simulink model "Grid_modelling_Thermal_V7_ALfix_sheddable_ramped"  (R2025b)
settings: Solver=ode45  StopTime=5000  MaxStep=0.01
libraries: simulink x20, slpidlib x10
(part 1 of 3)
settings Model: Creator=ASUS  LastModifiedBy=naren

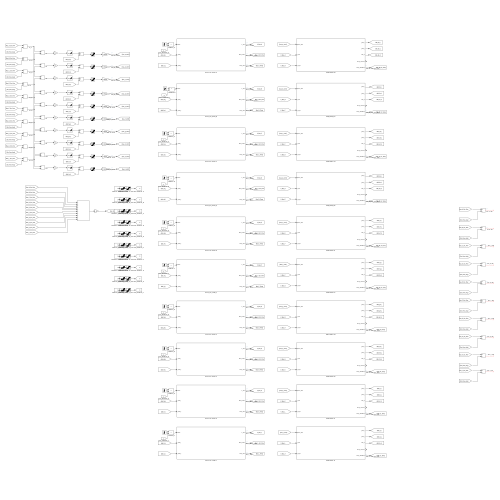
[thumbnail: Simulink's stored preview of the top-level diagram]
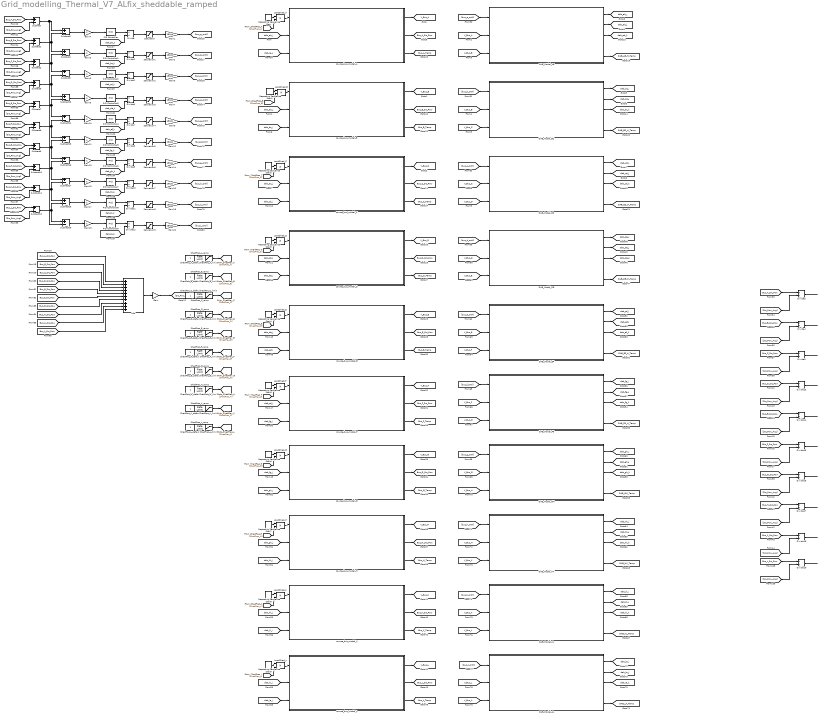
== system Grid_modelling_Thermal_V7_ALfix_sheddable_ramped ==
  Add : Sum  Inputs=++++++++++
  DAB_Model_AB : Subsystem
  DAB_Model_AL : Subsystem
  DAB_Model_BC : Subsystem
  DAB_Model_CD : Subsystem
  DAB_Model_DE : Subsystem
  DAB_Model_EF : Subsystem
  DAB_Model_FG : Subsystem
  DAB_Model_GH : Subsystem
  DAB_Model_HK : Subsystem
  DAB_Model_KL : Subsystem
  Divide{,1..19} (20 alike) : Product  Inputs=*/
  Gain : Gain  Gain=1/10
  Gain{1..3,7,9,12,14,16,18,20} (10 alike) : Gain  Gain=180/pi
  Gain{4..6,8,10..11,13,15,17,19} (10 alike) : Gain  Gain=-1
  LoadShed_A : Product
  LoadShed_B : Product
  LoadShed_C : Product
  LoadShed_D : Product
  LoadShed_E : Product
  LoadShed_F : Product
  LoadShed_G : Product
  LoadShed_H : Product
  LoadShed_K : Product
  LoadShed_L : Product
  PID Controller{,1..9} (10 alike) : slpidlib/PID Controller  Controller=PI  Form=Parallel  TimeDomain=Discrete-time  UseExternalTs=off  SampleTime=0.01  IntegratorMethod=Forward Euler  FilterMethod=Forward Euler  ControllerParametersSource=internal  P=0.2  I=0.1  UseKiTs=off  D=0  UseExternalDerivativeSource=off  N=100  UseFilter=on  TunerSelectOption=Transfer Function Based (PID Tuner App)  InitialConditionSource=internal  InitialConditionForIntegrator=0  InitialConditionForFilter=0  DifferentiatorICPrevScaledInput=0  ExternalReset=none  TrackingMode=off  Kt=1  LimitOutput=on  SatLimitsSource=internal  UpperSaturationLimit=100e3  LowerSaturationLimit=-100e3  LinearizeAsGain=on  AntiWindupMode=none  Kb=1  LimitIntegrator=off  UpperIntegratorSaturationLimit=inf  LowerIntegratorSaturationLimit=-inf  POutMin=[]  POutMax=[]  IOutMin=[]  IOutMax=[]  DOutMin=[]  DOutMax=[]  NOutMin=[]  NOutMax=[]  SumOutMin=[]  SumOutMax=[]  SaturationOutMin=[]  SaturationOutMax=[]  PParamMin=[]  PParamMax=[]  IParamMin=[]  IParamMax=[]  DParamMin=[]  DParamMax=[]  NParamMin=[]  NParamMax=[]  KbParamMin=[]  KbParamMax=[]  KtParamMin=[]  KtParamMax=[]  KbOutMin=[]  KbOutMax=[]  KtOutMin=[]  KtOutMax=[]  IntegratorOutMin=[]  IntegratorOutMax=[]  FilterOutMin=[]  FilterOutMax=[]  SumI1OutMin=[]  SumI1OutMax=[]  SumI2OutMin=[]  SumI2OutMax=[]  SumI3OutMin=[]  SumI3OutMax=[]  SumI4OutMin=[]  SumI4OutMax=[]  SumDOutMin=[]  SumDOutMax=[]  DifferentiatorOutMin=[]  DifferentiatorOutMax=[]  FilterDiffOutCoefMin=[]  FilterDiffOutCoefMax=[]  ReciprocalOutMin=[]  ReciprocalOutMax=[]  SumDenOutMin=[]  SumDenOutMax=[]  SumNumOutMin=[]  SumNumOutMax=[]  DivideOutMin=[]  DivideOutMax=[]  UdiffTsProdOutMin=[]  UdiffTsProdOutMax=[]  NTsProdOutMin=[]  NTsProdOutMax=[]  UintegralTsProdOutMin=[]  UintegralTsProdOutMax=[]  UngainTsProdOutMin=[]  UngainTsProdOutMax=[]  ClampingZeroOutDataTypeStr=Inherit: Inherit via back propagation  ClampingZeroOutMin=[]  ClampingZeroOutMax=[]  FilterDenConstantOutDataTypeStr=Inherit: Inherit via back propagation  FilterDenConstantOutMin=[]  FilterDenConstantOutMax=[]  PCopyOutDataTypeStr=Inherit: Inherit via back propagation  PCopyOutMin=[]  PCopyOutMax=[]  NCopyOutDataTypeStr=Inherit: Inherit via back propagation  NCopyOutMin=[]  NCopyOutMax=[]  IntegratorContinuousStateAttributes=''  IntegratorStateMustResolveToSignalObject=off  IntegratorRTWStateStorageClass=Auto  FilterContinuousStateAttributes=''  FilterStateMustResolveToSignalObject=off  FilterRTWStateStorageClass=Auto  ParallelPVariant=InternalParameters  IdealPVariant=Disabled  IVariant=InternalParameters  DVariant=Disabled  IntegratorVariant=Discrete  SatVariant=Enabled  AWVariant=Passthrough  PCopyVariant=Disabled  TRVariant=Disabled  FdbkBlocksVariant=Forward  IdealPFdbkVariant=Disabled  SatFdbkVariant=Disabled  DerivativeFilterVariant=Disabled  NVariant=Disabled  NCopyVariant=Disabled_SignalSpec  FilterICVariant=Disabled  IntegratorICVariant=InternalICs  ExternalResetVariant=Disabled  TRSumVariant=Passthrough  SumFdbkVariant=Disabled  SumVariant=Sum_PI  TsampFilterVariant=InternalTs  TsampNgainVariant=Passthrough  TsampIntegralVariant=Disabled_SignalSpec  ExternalSaturationOutDataTypeStr=Inherit: Same as second input  DerivativeSourceVariant=Disabled  PreIntVariant=InternalPreInt
  Repeating Sequence Stair : simulink/Sources/Repeating Sequence Stair  OutValues=Pload_A.'  tsamp=0.01  OutMin=[]  OutMax=[]  OutDataTypeStr=double  OutputDataTypeScalingMode=double  OutDataType=fixdt(0,8)  ConRadixGroup=Best Precision: Vector-wise  OutScaling=2^-12
  Repeating Sequence Stair1 : simulink/Sources/Repeating Sequence Stair  OutValues=Pload_B.'  tsamp=0.01  OutMin=[]  OutMax=[]  OutDataTypeStr=double  OutputDataTypeScalingMode=double  OutDataType=fixdt(0,8)  ConRadixGroup=Best Precision: Vector-wise  OutScaling=2^-12
  Repeating Sequence Stair2 : simulink/Sources/Repeating Sequence Stair  OutValues=Pload_C.'  tsamp=0.01  OutMin=[]  OutMax=[]  OutDataTypeStr=double  OutputDataTypeScalingMode=double  OutDataType=fixdt(0,8)  ConRadixGroup=Best Precision: Vector-wise  OutScaling=2^-12
  Repeating Sequence Stair3 : simulink/Sources/Repeating Sequence Stair  OutValues=Pload_D.'  tsamp=0.01  OutMin=[]  OutMax=[]  OutDataTypeStr=double  OutputDataTypeScalingMode=double  OutDataType=fixdt(0,8)  ConRadixGroup=Best Precision: Vector-wise  OutScaling=2^-12
  Repeating Sequence Stair4 : simulink/Sources/Repeating Sequence Stair  OutValues=Pload_E.'  tsamp=0.01  OutMin=[]  OutMax=[]  OutDataTypeStr=double  OutputDataTypeScalingMode=double  OutDataType=fixdt(0,8)  ConRadixGroup=Best Precision: Vector-wise  OutScaling=2^-12
  Repeating Sequence Stair5 : simulink/Sources/Repeating Sequence Stair  OutValues=Pload_F.'  tsamp=0.01  OutMin=[]  OutMax=[]  OutDataTypeStr=double  OutputDataTypeScalingMode=double  OutDataType=fixdt(0,8)  ConRadixGroup=Best Precision: Vector-wise  OutScaling=2^-12
  Repeating Sequence Stair6 : simulink/Sources/Repeating Sequence Stair  OutValues=Pload_G.'  tsamp=0.01  OutMin=[]  OutMax=[]  OutDataTypeStr=double  OutputDataTypeScalingMode=double  OutDataType=fixdt(0,8)  ConRadixGroup=Best Precision: Vector-wise  OutScaling=2^-12
  Repeating Sequence Stair7 : simulink/Sources/Repeating Sequence Stair  OutValues=Pload_H.'  tsamp=0.01  OutMin=[]  OutMax=[]  OutDataTypeStr=double  OutputDataTypeScalingMode=double  OutDataType=fixdt(0,8)  ConRadixGroup=Best Precision: Vector-wise  OutScaling=2^-12
  Repeating Sequence Stair8 : simulink/Sources/Repeating Sequence Stair  OutValues=Pload_K.'  tsamp=0.01  OutMin=[]  OutMax=[]  OutDataTypeStr=double  OutputDataTypeScalingMode=double  OutDataType=fixdt(0,8)  ConRadixGroup=Best Precision: Vector-wise  OutScaling=2^-12
  Repeating Sequence Stair9 : simulink/Sources/Repeating Sequence Stair  OutValues=Pload_L.'  tsamp=0.01  OutMin=[]  OutMax=[]  OutDataTypeStr=double  OutputDataTypeScalingMode=double  OutDataType=fixdt(0,8)  ConRadixGroup=Best Precision: Vector-wise  OutScaling=2^-12
  Saturation{,1..9} (10 alike) : Saturate  UpperLimit=pi/2  LowerLimit=-pi/2
  ShedFrac_A_default : Constant
  ShedFrac_A_limit : Saturate  UpperLimit=1  LowerLimit=0
  ShedFrac_A_ramp : RateLimiter  RisingSlewLimit=inf  FallingSlewLimit=-inf  SampleTimeMode=inherited
  ShedFrac_B_default : Constant
  ShedFrac_B_limit : Saturate  UpperLimit=1  LowerLimit=0
  ShedFrac_B_ramp : RateLimiter  RisingSlewLimit=inf  FallingSlewLimit=-inf  SampleTimeMode=inherited
  ShedFrac_C_default : Constant
  ShedFrac_C_limit : Saturate  UpperLimit=1  LowerLimit=0
  ShedFrac_C_ramp : RateLimiter  RisingSlewLimit=inf  FallingSlewLimit=-inf  SampleTimeMode=inherited
  ShedFrac_D_default : Constant
  ShedFrac_D_limit : Saturate  UpperLimit=1  LowerLimit=0
  ShedFrac_D_ramp : RateLimiter  RisingSlewLimit=inf  FallingSlewLimit=-inf  SampleTimeMode=inherited
  ShedFrac_E_default : Constant
  ShedFrac_E_limit : Saturate  UpperLimit=1  LowerLimit=0
  ShedFrac_E_ramp : RateLimiter  RisingSlewLimit=inf  FallingSlewLimit=-inf  SampleTimeMode=inherited
  ShedFrac_F_default : Constant
  ShedFrac_F_limit : Saturate  UpperLimit=1  LowerLimit=0
  ShedFrac_F_ramp : RateLimiter  RisingSlewLimit=inf  FallingSlewLimit=-inf  SampleTimeMode=inherited
  ShedFrac_G_default : Constant
  ShedFrac_G_limit : Saturate  UpperLimit=1  LowerLimit=0
  ShedFrac_G_ramp : RateLimiter  RisingSlewLimit=inf  FallingSlewLimit=-inf  SampleTimeMode=inherited
  ShedFrac_H_default : Constant
  ShedFrac_H_limit : Saturate  UpperLimit=1  LowerLimit=0
  ShedFrac_H_ramp : RateLimiter  RisingSlewLimit=inf  FallingSlewLimit=-inf  SampleTimeMode=inherited
  ShedFrac_K_default : Constant
  ShedFrac_K_limit : Saturate  UpperLimit=1  LowerLimit=0
  ShedFrac_K_ramp : RateLimiter  RisingSlewLimit=inf  FallingSlewLimit=-inf  SampleTimeMode=inherited
  ShedFrac_L_default : Constant
  ShedFrac_L_limit : Saturate  UpperLimit=1  LowerLimit=0
  ShedFrac_L_ramp : RateLimiter  RisingSlewLimit=inf  FallingSlewLimit=-inf  SampleTimeMode=inherited
  Subtract{,1..19} (20 alike) : Sum  Inputs=+-
  source_bus_model_A : Subsystem
  source_bus_model_B : Subsystem
  source_bus_model_C : Subsystem
  source_bus_model_D : Subsystem
  source_bus_model_E : Subsystem
  source_bus_model_F : Subsystem
  source_bus_model_G : Subsystem
  source_bus_model_H : Subsystem
  source_bus_model_K : Subsystem
  source_bus_model_L : Subsystem
  tag scope: Bus_A_Src_Pow=global, Bus_A_Temp=global, Bus_B_Src_Pow=global, Bus_B_Temp=global, Bus_C_Src_Pow=global, Bus_C_Temp=global, Bus_D_Src_Pow=global, Bus_D_Temp=global, Bus_E_Src_Pow=global, Bus_E_Temp=global, Bus_F_Src_Pow=global, Bus_F_Temp=global, Bus_G_Src_Pow=global, Bus_G_Temp=global, Bus_H_Src_Pow=global, Bus_H_Temp=global, Bus_K_Src_Pow=global, Bus_K_Temp=global, Bus_L_Src_Pow=global, Bus_L_Temp=global, DAB_AB_H_Temp=global, DAB_BC_H_Temp=global, DAB_CD_H_Temp=global, DAB_DE_H_Temp=global, DAB_EF_H_Temp=global, DAB_FG_H_Temp=global, DAB_GH_Temp=global, DAB_HK_Temp=global, DAB_KL_Temp=global, DAB_LA_Temp=global, V_Bus_A=global, V_Bus_B=global, V_Bus_C=global, V_Bus_D=global, V_Bus_E=global, V_Bus_F=global, V_Bus_G=global, V_Bus_H=global, V_Bus_K=global, V_Bus_L=global, dab_ab_i=global, dab_ab_j=global, dab_ab_k=global, dab_bc_i=global, dab_bc_j=global, dab_bc_k=global, dab_cd_i=global, dab_cd_j=global, dab_cd_k=global, dab_de_i=global, dab_de_j=global, dab_de_k=global, dab_ef_i=global, dab_ef_j=global, dab_ef_k=global, dab_fg_i=global, dab_fg_j=global, dab_fg_k=global, dab_gh_i=global, dab_gh_j=global, dab_gh_k=global, dab_hk_i=global, dab_hk_j=global, dab_hk_k=global, dab_kl_i=global, dab_kl_j=global, dab_kl_k=global, dab_la_i=global, dab_la_j=global, dab_la_k=global
  wires:
  source_bus_model_B/1(V_bus) -> [V_Bus_B]  "Bus_B_Voltage"
  source_bus_model_C/1(V_bus) -> [V_Bus_C]  "Bus_C_Voltage"
  source_bus_model_A/1(V_bus) -> [V_Bus_A]  "Bus_A_Voltage"
  DAB_Model_AB/1(i_dab_i) -> [dab_ab_i]
  DAB_Model_AB/2(i_dab_j) -> [dab_ab_j]
  DAB_Model_BC/1(i_dab_i) -> [dab_bc_i]
  DAB_Model_BC/2(i_dab_j) -> [dab_bc_j]
  DAB_Model_CD/1(i_dab_i) -> [dab_cd_i]
  DAB_Model_CD/2(i_dab_j) -> [dab_cd_j]
  [dab_ab_i] -> source_bus_model_A/2(i_dab_1)
  [dab_ab_j] -> source_bus_model_B/2(i_dab_1)
  [V_Bus_A] -> DAB_Model_AB/2(v_left)
  [V_Bus_B] -> DAB_Model_AB/3(v_right)
  [V_Bus_B] -> DAB_Model_BC/2(v_left)
  [V_Bus_C] -> DAB_Model_BC/3(v_right)
  [dab_bc_i] -> source_bus_model_B/3(i_dab_2)
  [dab_bc_j] -> source_bus_model_C/2(i_dab_1)
  [V_Bus_C] -> DAB_Model_CD/2(v_left)
  [V_Bus_D] -> DAB_Model_CD/3(v_right)
  [dab_la_j] -> source_bus_model_A/3(i_dab_2)
  [dab_cd_i] -> source_bus_model_C/3(i_dab_2)
  [bus_a_cntrl] -> DAB_Model_AB/1(phase_shift)
  [bus_b_cntrl] -> DAB_Model_BC/1(phase_shift)
  [bus_c_cntrl] -> DAB_Model_CD/1(phase_shift)
  source_bus_model_A/2(Bus_Power) -> [Bus_A_Src_Pow]  "Bus_A_Source_Power"
  source_bus_model_B/2(Bus_Power) -> [Bus_B_Src_Pow]  "Bus_B_Source_Power"
  source_bus_model_C/2(Bus_Power) -> [Bus_C_Src_Pow]  "Bus_C_Source_Power"
  [Bus_A_Src_Pow] -> Add/1
  [Bus_C_Src_Pow] -> Add/3
  [Bus_B_Src_Pow] -> Add/2
  Add/1 -> Gain/1
  Gain/1 -> [Src_Pow_Avg]
  [Src_Pow_Avg] -> Subtract/2
  [Bus_A_Src_Pow] -> Subtract/1
  [Bus_B_Src_Pow] -> Subtract1/1
  [Src_Pow_Avg] -> Subtract1/2
  [Bus_C_Src_Pow] -> Subtract2/1
  [Src_Pow_Avg] -> Subtract2/2
  Subtract1/1 -> Subtract4/1, Subtract3/2  "del_p2"
  Subtract2/1 -> Subtract4/2, Subtract5/1  "del_p3"
  Subtract3/1 -> Gain4/1  "e12"
  Subtract4/1 -> Gain5/1  "e23"
  Subtract5/1 -> Gain6/1  "e34"
  DAB_Model_AB/3(dab_k) -> [dab_ab_k]
  DAB_Model_BC/3(dab_k) -> [dab_bc_k]
  DAB_Model_CD/3(dab_k) -> [dab_cd_k]
  PID Controller/1 -> Divide/1
  PID Controller1/1 -> Divide1/1
  PID Controller2/1 -> Divide2/1
  [dab_ab_k] -> Divide/2
  [dab_bc_k] -> Divide1/2
  [dab_cd_k] -> Divide2/2
  Divide/1 -> Saturation/1
  Divide1/1 -> Saturation1/1
  Divide2/1 -> Saturation2/1
  Saturation/1 -> Gain1/1
  Saturation1/1 -> Gain2/1
  Saturation2/1 -> Gain3/1
  Gain1/1 -> [bus_a_cntrl]  "DAB_AB_Phase"
  Gain2/1 -> [bus_b_cntrl]  "DAB_BC_Phase"
  Gain3/1 -> [bus_c_cntrl]  "DAB_AC_Phase"
  Gain4/1 -> PID Controller/1
  Gain5/1 -> PID Controller1/1
  Gain6/1 -> PID Controller2/1
  [Bus_A_Src_Pow] -> Divide3/1
  [Src_Pow_Avg] -> Divide3/2
  [Src_Pow_Avg] -> Divide4/2
  [Bus_B_Src_Pow] -> Divide4/1
  [Src_Pow_Avg] -> Divide5/2
  [Bus_C_Src_Pow] -> Divide5/1
  Divide4/1 -> ?  "Bus_B_GEI"
  Divide3/1 -> ?  "Bus_A_GEI"
  Divide5/1 -> ?  "Bus_C_GEI"
  DAB_Model_AB/5(Temp_HeatSink) -> [DAB_AB_H_Temp]  "DAB_AB_Heat_Sink_Temp"
  DAB_Model_BC/5(Temp_HeatSink) -> [DAB_BC_H_Temp]  "DAB_BC_Heat_Sink_Temp"
  DAB_Model_CD/5(Temp_HeatSink) -> [DAB_CD_H_Temp]  "DAB_CD_Heat_Sink_Temp"
  source_bus_model_B/3(Temp_bus) -> [Bus_B_Temp]  "Bus_B_Temp"
  source_bus_model_A/3(Temp_bus) -> [Bus_A_Temp]  "Bus_A_Temp"
  source_bus_model_C/3(Temp_bus) -> [Bus_C_Temp]  "Bus_C_Temp"
  [dab_de_i] -> source_bus_model_D/3(i_dab_2)
  source_bus_model_D/3(Temp_bus) -> [Bus_D_Temp]  "Bus_D_Temp"
  source_bus_model_D/1(V_bus) -> [V_Bus_D]  "Bus_D_Voltage"
  [dab_cd_j] -> source_bus_model_D/2(i_dab_1)
  source_bus_model_D/2(Bus_Power) -> [Bus_D_Src_Pow]  "Bus_D_Source_Power"
  source_bus_model_E/1(V_bus) -> [V_Bus_E]  "Bus_E_Voltage"
  source_bus_model_E/2(Bus_Power) -> [Bus_E_Src_Pow]  "Bus_E_Source_Power"
  [dab_de_j] -> source_bus_model_E/2(i_dab_1)
  [dab_ef_i] -> source_bus_model_E/3(i_dab_2)
  source_bus_model_E/3(Temp_bus) -> [Bus_E_Temp]  "Bus_E_Temp"
  [dab_ef_j] -> source_bus_model_F/2(i_dab_1)
  source_bus_model_F/2(Bus_Power) -> [Bus_F_Src_Pow]  "Bus_F_Source_Power"
  source_bus_model_F/1(V_bus) -> [V_Bus_F]  "Bus_F_Voltage"
  source_bus_model_F/3(Temp_bus) -> [Bus_F_Temp]  "Bus_F_Temp"
  [dab_fg_i] -> source_bus_model_F/3(i_dab_2)
  [dab_gh_i] -> source_bus_model_G/3(i_dab_2)
  source_bus_model_G/3(Temp_bus) -> [Bus_G_Temp]  "Bus_G_Temp"
  [dab_fg_j] -> source_bus_model_G/2(i_dab_1)
  source_bus_model_G/1(V_bus) -> [V_Bus_G]  "Bus_G_Voltage"
  source_bus_model_G/2(Bus_Power) -> [Bus_G_Src_Pow]  "Bus_G_Source_Power"
  source_bus_model_H/2(Bus_Power) -> [Bus_H_Src_Pow]  "Bus_H_Source_Power"
  [dab_hk_i] -> source_bus_model_H/3(i_dab_2)
  [dab_gh_j] -> source_bus_model_H/2(i_dab_1)
  source_bus_model_H/3(Temp_bus) -> [Bus_H_Temp]  "Bus_H_Temp"
  source_bus_model_H/1(V_bus) -> [V_Bus_H]  "Bus_H_Voltage"
  source_bus_model_K/1(V_bus) -> [V_Bus_K]  "Bus_K_Voltage"
  [dab_hk_j] -> source_bus_model_K/2(i_dab_1)
  source_bus_model_K/2(Bus_Power) -> [Bus_K_Src_Pow]  "Bus_K_Source_Power"
  [dab_kl_i] -> source_bus_model_K/3(i_dab_2)
  source_bus_model_K/3(Temp_bus) -> [Bus_K_Temp]  "Bus_K_Temp"
  [dab_la_i] -> source_bus_model_L/3(i_dab_2)
  [dab_kl_j] -> source_bus_model_L/2(i_dab_1)
  source_bus_model_L/2(Bus_Power) -> [Bus_L_Src_Pow]  "Bus_L_Source_Power"
  source_bus_model_L/3(Temp_bus) -> [Bus_L_Temp]  "Bus_L_Temp"
  source_bus_model_L/1(V_bus) -> [V_Bus_L]  "Bus_L_Voltage"
  [V_Bus_E] -> DAB_Model_DE/3(v_right)
  DAB_Model_DE/1(i_dab_i) -> [dab_de_i]
  DAB_Model_DE/5(Temp_HeatSink) -> [DAB_DE_H_Temp]  "DAB_DE_Heat_Sink_Temp"
  DAB_Model_DE/2(i_dab_j) -> [dab_de_j]
  [bus_d_cntrl] -> DAB_Model_DE/1(phase_shift)
  [V_Bus_D] -> DAB_Model_DE/2(v_left)
  DAB_Model_DE/3(dab_k) -> [dab_de_k]
  [V_Bus_E] -> DAB_Model_EF/2(v_left)
  DAB_Model_EF/3(dab_k) -> [dab_ef_k]
  [bus_e_cntrl] -> DAB_Model_EF/1(phase_shift)
  DAB_Model_EF/2(i_dab_j) -> [dab_ef_j]
  DAB_Model_EF/1(i_dab_i) -> [dab_ef_i]
  DAB_Model_EF/5(Temp_HeatSink) -> [DAB_EF_H_Temp]  "DAB_EF_Heat_Sink_Temp"
  [V_Bus_F] -> DAB_Model_EF/3(v_right)
  DAB_Model_FG/5(Temp_HeatSink) -> [DAB_FG_H_Temp]  "DAB_FG_Heat_Sink_Temp"
  [V_Bus_F] -> DAB_Model_FG/2(v_left)
  DAB_Model_FG/1(i_dab_i) -> [dab_fg_i]
  [bus_f_cntrl] -> DAB_Model_FG/1(phase_shift)
  DAB_Model_FG/2(i_dab_j) -> [dab_fg_j]
  DAB_Model_FG/3(dab_k) -> [dab_fg_k]
  [V_Bus_G] -> DAB_Model_FG/3(v_right)
  [V_Bus_H] -> DAB_Model_GH/3(v_right)
  DAB_Model_GH/2(i_dab_j) -> [dab_gh_j]
  DAB_Model_GH/3(dab_k) -> [dab_gh_k]
  [bus_g_cntrl] -> DAB_Model_GH/1(phase_shift)
  DAB_Model_GH/1(i_dab_i) -> [dab_gh_i]
  DAB_Model_GH/5(Temp_HeatSink) -> [DAB_GH_Temp]  "DAB_GH_Heat_Sink_Temp"
  [V_Bus_G] -> DAB_Model_GH/2(v_left)
  DAB_Model_HK/3(dab_k) -> [dab_hk_k]
  [V_Bus_H] -> DAB_Model_HK/2(v_left)
  DAB_Model_HK/5(Temp_HeatSink) -> [DAB_HK_Temp]  "DAB_HK_Heat_Sink_Temp"
  DAB_Model_HK/1(i_dab_i) -> [dab_hk_i]
  [bus_h_cntrl] -> DAB_Model_HK/1(phase_shift)
  DAB_Model_HK/2(i_dab_j) -> [dab_hk_j]
  [V_Bus_K] -> DAB_Model_HK/3(v_right)
  [V_Bus_K] -> DAB_Model_KL/2(v_left)
  DAB_Model_KL/2(i_dab_j) -> [dab_kl_j]
  [bus_k_cntrl] -> DAB_Model_KL/1(phase_shift)
  DAB_Model_KL/1(i_dab_i) -> [dab_kl_i]
  DAB_Model_KL/5(Temp_HeatSink) -> [DAB_KL_Temp]  "DAB_KL_Heat_Sink_Temp"
  [V_Bus_L] -> DAB_Model_KL/3(v_right)
  DAB_Model_KL/3(dab_k) -> [dab_kl_k]
  [V_Bus_L] -> DAB_Model_AL/2(v_left)
  DAB_Model_AL/3(dab_k) -> [dab_la_k]
  [V_Bus_A] -> DAB_Model_AL/3(v_right)
  DAB_Model_AL/2(i_dab_j) -> [dab_la_j]
  DAB_Model_AL/1(i_dab_i) -> [dab_la_i]
  DAB_Model_AL/5(Temp_HeatSink) -> [DAB_LA_Temp]  "DAB_LA_Heat_Sink_Temp"
  [bus_l_cntrl] -> DAB_Model_AL/1(phase_shift)
  [Bus_D_Src_Pow] -> Add/4
  [Bus_E_Src_Pow] -> Add/5
  [Bus_F_Src_Pow] -> Add/6
  [Bus_G_Src_Pow] -> Add/7
  [Bus_H_Src_Pow] -> Add/8
  [Bus_K_Src_Pow] -> Add/9
  [Bus_L_Src_Pow] -> Add/10
  [Src_Pow_Avg] -> Subtract6/2
  [Bus_D_Src_Pow] -> Subtract6/1
  Subtract7/1 -> Subtract13/2, Subtract14/1  "del_p5"
  [Bus_E_Src_Pow] -> Subtract7/1
  [Src_Pow_Avg] -> Subtract7/2
  [Bus_F_Src_Pow] -> Subtract8/1
  [Src_Pow_Avg] -> Subtract8/2
  Subtract8/1 -> Subtract14/2, Subtract15/1  "del_p6"
  Subtract9/1 -> Subtract15/2, Subtract16/1  "del_p7"
  [Src_Pow_Avg] -> Subtract9/2
  [Bus_G_Src_Pow] -> Subtract9/1
  [Bus_H_Src_Pow] -> Subtract10/1
  Subtract10/1 -> Subtract16/2, Subtract17/1  "del_p8"
  [Src_Pow_Avg] -> Subtract10/2
  Subtract11/1 -> Subtract17/2, Subtract18/1  "del_p9"
  [Src_Pow_Avg] -> Subtract11/2
  [Bus_K_Src_Pow] -> Subtract11/1
  [Src_Pow_Avg] -> Subtract12/2
  Subtract12/1 -> Subtract18/2, Subtract19/1  "del_p10"
  [Bus_L_Src_Pow] -> Subtract12/1
  Gain7/1 -> [bus_d_cntrl]  "DAB_DE_Phase"
  Gain8/1 -> PID Controller3/1
  [dab_de_k] -> Divide6/2
  Subtract/1 -> Subtract19/2, Subtract3/1  "del_p1"
  Divide6/1 -> Saturation3/1
  Subtract13/1 -> Gain8/1  "e45"
  PID Controller3/1 -> Divide6/1
  Saturation3/1 -> Gain7/1
  Subtract6/1 -> Subtract5/2, Subtract13/1  "del_p4"
  PID Controller4/1 -> Divide7/1
  Divide7/1 -> Saturation4/1
  Gain10/1 -> PID Controller4/1
  Gain9/1 -> [bus_e_cntrl]  "DAB_EF_Phase"
  Saturation4/1 -> Gain9/1
  [dab_ef_k] -> Divide7/2
  Subtract14/1 -> Gain10/1  "e56"
  Saturation5/1 -> Gain12/1
  Divide8/1 -> Saturation5/1
  Gain12/1 -> [bus_f_cntrl]  "DAB_FG_Phase"
  Gain11/1 -> PID Controller5/1
  Subtract15/1 -> Gain11/1  "e67"
  PID Controller5/1 -> Divide8/1
  [dab_fg_k] -> Divide8/2
  Subtract16/1 -> Gain13/1  "e78"
  Saturation6/1 -> Gain14/1
  Gain13/1 -> PID Controller6/1
  Divide9/1 -> Saturation6/1
  [dab_gh_k] -> Divide9/2
  Gain14/1 -> [bus_g_cntrl]  "DAB_GH_Phase"
  PID Controller6/1 -> Divide9/1
  Subtract17/1 -> Gain15/1  "e89"
  PID Controller7/1 -> Divide10/1
  Saturation7/1 -> Gain16/1
  [dab_hk_k] -> Divide10/2
  Gain16/1 -> [bus_h_cntrl]  "DAB_HK_Phase"
  Divide10/1 -> Saturation7/1
  Gain15/1 -> PID Controller7/1
  Gain17/1 -> PID Controller8/1
  [dab_kl_k] -> Divide11/2
  Saturation8/1 -> Gain18/1
  Subtract18/1 -> Gain17/1  "e910"
  Gain18/1 -> [bus_k_cntrl]  "DAB_KL_Phase"
  PID Controller8/1 -> Divide11/1
  Divide11/1 -> Saturation8/1
  Saturation9/1 -> Gain20/1
  [dab_la_k] -> Divide12/2
  Subtract19/1 -> Gain19/1  "e101"
  Gain20/1 -> [bus_l_cntrl]  "DAB_LA_Phase"
  Divide12/1 -> Saturation9/1
  Gain19/1 -> PID Controller9/1
  PID Controller9/1 -> Divide12/1
  [Bus_D_Src_Pow] -> Divide13/1
  [Src_Pow_Avg] -> Divide13/2
  Divide13/1 -> ?  "Bus_D_GEI"
  [Src_Pow_Avg] -> Divide14/2
  Divide14/1 -> ?  "Bus_E_GEI"
  [Bus_E_Src_Pow] -> Divide14/1
  Divide15/1 -> ?  "Bus_F_GEI"
  [Src_Pow_Avg] -> Divide15/2
  [Bus_F_Src_Pow] -> Divide15/1
  [Src_Pow_Avg] -> Divide16/2
  [Bus_G_Src_Pow] -> Divide16/1
  Divide16/1 -> ?  "Bus_G_GEI"
  [Bus_H_Src_Pow] -> Divide17/1
  Divide17/1 -> ?  "Bus_H_GEI"
  [Src_Pow_Avg] -> Divide17/2
  [Src_Pow_Avg] -> Divide18/2
  [Bus_K_Src_Pow] -> Divide18/1
  Divide18/1 -> ?  "Bus_K_GEI"
  [Src_Pow_Avg] -> Divide19/2
  [Bus_L_Src_Pow] -> Divide19/1
  Divide19/1 -> ?  "Bus_L_GEI"
  ShedFrac_A_limit/1 -> [ShedFrac_A]
  Repeating Sequence Stair/1 -> LoadShed_A/1
  [ShedFrac_A] -> LoadShed_A/2
  LoadShed_A/1 -> source_bus_model_A/1(Pload)
  ShedFrac_B_limit/1 -> [ShedFrac_B]
  Repeating Sequence Stair1/1 -> LoadShed_B/1
  [ShedFrac_B] -> LoadShed_B/2
  LoadShed_B/1 -> source_bus_model_B/1(Pload)
  ShedFrac_C_limit/1 -> [ShedFrac_C]
  Repeating Sequence Stair2/1 -> LoadShed_C/1
  [ShedFrac_C] -> LoadShed_C/2
  LoadShed_C/1 -> source_bus_model_C/1(Pload)
  ShedFrac_D_limit/1 -> [ShedFrac_D]
  Repeating Sequence Stair3/1 -> LoadShed_D/1
  [ShedFrac_D] -> LoadShed_D/2
  LoadShed_D/1 -> source_bus_model_D/1(Pload)
  ShedFrac_E_limit/1 -> [ShedFrac_E]
  Repeating Sequence Stair4/1 -> LoadShed_E/1
  [ShedFrac_E] -> LoadShed_E/2
  LoadShed_E/1 -> source_bus_model_E/1(Pload)
  ShedFrac_F_limit/1 -> [ShedFrac_F]
  Repeating Sequence Stair5/1 -> LoadShed_F/1
  [ShedFrac_F] -> LoadShed_F/2
  LoadShed_F/1 -> source_bus_model_F/1(Pload)
  ShedFrac_G_limit/1 -> [ShedFrac_G]
  Repeating Sequence Stair6/1 -> LoadShed_G/1
  [ShedFrac_G] -> LoadShed_G/2
  LoadShed_G/1 -> source_bus_model_G/1(Pload)
  ShedFrac_H_limit/1 -> [ShedFrac_H]
  Repeating Sequence Stair7/1 -> LoadShed_H/1
  [ShedFrac_H] -> LoadShed_H/2
  LoadShed_H/1 -> source_bus_model_H/1(Pload)
  ShedFrac_K_limit/1 -> [ShedFrac_K]
  Repeating Sequence Stair8/1 -> LoadShed_K/1
  [ShedFrac_K] -> LoadShed_K/2
  LoadShed_K/1 -> source_bus_model_K/1(Pload)
  ShedFrac_L_limit/1 -> [ShedFrac_L]
  Repeating Sequence Stair9/1 -> LoadShed_L/1
  [ShedFrac_L] -> LoadShed_L/2
  LoadShed_L/1 -> source_bus_model_L/1(Pload)
  ShedFrac_A_default/1 -> ShedFrac_A_ramp/1
  ShedFrac_A_ramp/1 -> ShedFrac_A_limit/1
  ShedFrac_B_default/1 -> ShedFrac_B_ramp/1
  ShedFrac_B_ramp/1 -> ShedFrac_B_limit/1
  ShedFrac_C_default/1 -> ShedFrac_C_ramp/1
  ShedFrac_C_ramp/1 -> ShedFrac_C_limit/1
  ShedFrac_D_default/1 -> ShedFrac_D_ramp/1
  ShedFrac_D_ramp/1 -> ShedFrac_D_limit/1
  ShedFrac_E_default/1 -> ShedFrac_E_ramp/1
  ShedFrac_E_ramp/1 -> ShedFrac_E_limit/1
  ShedFrac_F_default/1 -> ShedFrac_F_ramp/1
  ShedFrac_F_ramp/1 -> ShedFrac_F_limit/1
  ShedFrac_G_default/1 -> ShedFrac_G_ramp/1
  ShedFrac_G_ramp/1 -> ShedFrac_G_limit/1
  ShedFrac_H_default/1 -> ShedFrac_H_ramp/1
  ShedFrac_H_ramp/1 -> ShedFrac_H_limit/1
  ShedFrac_K_default/1 -> ShedFrac_K_ramp/1
  ShedFrac_K_ramp/1 -> ShedFrac_K_limit/1
  ShedFrac_L_default/1 -> ShedFrac_L_ramp/1
  ShedFrac_L_ramp/1 -> ShedFrac_L_limit/1

== system Grid_modelling_Thermal_V7_ALfix_sheddable_ramped/DAB_Model_AB ==
  phase_shift : Inport
  v_left : Inport  Port=2
  v_right : Inport  Port=3
  1/2*pi*fs : Gain  Gain=1 / (2*pi*10e3)
  1/Lk : Gain  Gain=1 / 340e-6
  Abs : Abs  SaturateOnIntegerOverflow=off
  Add Constant : Bias  Bias=1  SaturateOnIntegerOverflow=off
  Constant : Constant  Value=10
  DAB_Thermal_Model : Subsystem
  Divide : Product  Inputs=*/
  Divide1 : Product  Inputs=*/
  Gain : Gain  Gain=-1/pi
  Gain1 : Gain  Gain=-1
  Max : MinMax  Function=max  Inputs=2
  Max1 : MinMax  Function=max  Inputs=2
  Product : Product
  Product1 : Product  Inputs=3
  Saturation : Saturate  UpperLimit=pi/2  LowerLimit=-pi/2
  Saturation Dynamic : simulink/Discontinuities/Saturation Dynamic  OutMin=[]  OutMax=[]  OutDataTypeStr=Inherit: Same as second input  OutDataType=fixdt(1, 16)  OutScaling=2^-10  DoSatur=off
  Scope : Scope  NumInputPorts=2
      settings: ActiveDisplayYMinimum=8.97015  ActiveDisplayYMaximum=169.26864
  deg_2_rad : Gain  Gain=pi / 180
  thermal_derater : Subsystem
  turns_ratio : Gain  Gain=24/15
  i_dab_i : Outport
  i_dab_j : Outport  Port=2
  dab_k : Outport  Port=3
  Temp_Junction : Outport  Port=4
  Temp_HeatSink : Outport  Port=5
  wires:
  v_left/1 -> DAB_Thermal_Model/2(Va), Max/1, Product/1
  Constant/1 -> Max/2, Max1/2
  Add Constant/1 -> Product1/2
  Divide/1 -> Gain1/1
  v_right/1 -> DAB_Thermal_Model/3(Vb), Product/2, Max1/1
  Max1/1 -> Divide1/2
  Gain1/1 -> i_dab_i/1
  Divide1/1 -> i_dab_j/1
  Saturation/1 -> Product1/1, Abs/1
  1/2*pi*fs/1 -> 1/Lk/1
  phase_shift/1 -> deg_2_rad/1
  Gain/1 -> Add Constant/1
  1/Lk/1 -> dab_k/1, Product1/3
  Product/1 -> turns_ratio/1
  turns_ratio/1 -> 1/2*pi*fs/1
  Abs/1 -> Gain/1
  deg_2_rad/1 -> Saturation/1
  Max/1 -> Divide/2
  DAB_Thermal_Model/1(T_j) -> thermal_derater/1(Tj), Scope/1, Temp_Junction/1
  DAB_Thermal_Model/2(T_h) -> Temp_HeatSink/1
  Saturation Dynamic/1 -> DAB_Thermal_Model/1(P_ij), Divide1/1, Divide/1
  Product1/1 -> Saturation Dynamic/2  "P_ij"
  thermal_derater/1(derate_pos) -> Saturation Dynamic/1, Scope/2
  thermal_derater/2(derate_neg) -> Saturation Dynamic/3

== system Grid_modelling_Thermal_V7_ALfix_sheddable_ramped/DAB_Model_AL ==
  phase_shift : Inport
  v_left : Inport  Port=2
  v_right : Inport  Port=3
  1/2*pi*fs : Gain  Gain=1 / (2*pi*10e3)
  1/Lk : Gain  Gain=1 / 340e-6
  Abs : Abs  SaturateOnIntegerOverflow=off
  Add Constant : Bias  Bias=1  SaturateOnIntegerOverflow=off
  Constant : Constant  Value=10
  DAB_Thermal_Model : Subsystem
  Divide : Product  Inputs=*/
  Divide1 : Product  Inputs=*/
  Gain : Gain  Gain=-1/pi
  Gain1 : Gain  Gain=-1
  Max : MinMax  Function=max  Inputs=2
  Max1 : MinMax  Function=max  Inputs=2
  Product : Product
  Product1 : Product  Inputs=3
  Saturation : Saturate  UpperLimit=pi/2  LowerLimit=-pi/2
  Saturation Dynamic : simulink/Discontinuities/Saturation Dynamic  OutMin=[]  OutMax=[]  OutDataTypeStr=Inherit: Same as second input  OutDataType=fixdt(1, 16)  OutScaling=2^-10  DoSatur=off
  deg_2_rad : Gain  Gain=pi / 180
  thermal_derater : Subsystem
  turns_ratio : Gain  Gain=24/15
  i_dab_i : Outport
  i_dab_j : Outport  Port=2
  dab_k : Outport  Port=3
  Temp_Junction : Outport  Port=4
  Temp_HeatSink : Outport  Port=5
  wires:
  Constant/1 -> Max/2, Max1/2
  Add Constant/1 -> Product1/2
  Divide/1 -> Gain1/1
  Max1/1 -> Divide1/2
  Gain1/1 -> i_dab_i/1
  Divide1/1 -> i_dab_j/1
  Saturation Dynamic/1 -> DAB_Thermal_Model/1(P_ij), Divide1/1, Divide/1
  Saturation/1 -> Product1/1, Abs/1
  1/2*pi*fs/1 -> 1/Lk/1
  phase_shift/1 -> deg_2_rad/1
  Gain/1 -> Add Constant/1
  1/Lk/1 -> dab_k/1, Product1/3
  Product/1 -> turns_ratio/1
  turns_ratio/1 -> 1/2*pi*fs/1
  Abs/1 -> Gain/1
  deg_2_rad/1 -> Saturation/1
  Max/1 -> Divide/2
  v_right/1 -> DAB_Thermal_Model/3(Vb), Product/2, Max1/1
  v_left/1 -> DAB_Thermal_Model/2(Va), Max/1, Product/1
  Product1/1 -> Saturation Dynamic/2  "P_ij"
  DAB_Thermal_Model/1(T_j) -> thermal_derater/1(Tj), Temp_Junction/1
  DAB_Thermal_Model/2(T_h) -> Temp_HeatSink/1
  thermal_derater/1(derate_pos) -> Saturation Dynamic/1
  thermal_derater/2(derate_neg) -> Saturation Dynamic/3

== system Grid_modelling_Thermal_V7_ALfix_sheddable_ramped/DAB_Model_BC ==
  phase_shift : Inport
  v_left : Inport  Port=2
  v_right : Inport  Port=3
  1/2*pi*fs : Gain  Gain=1 / (2*pi*10e3)
  1/Lk : Gain  Gain=1 / 340e-6
  Abs : Abs  SaturateOnIntegerOverflow=off
  Add Constant : Bias  Bias=1  SaturateOnIntegerOverflow=off
  Constant : Constant  Value=10
  DAB_Thermal_Model : Subsystem
  Divide : Product  Inputs=*/
  Divide1 : Product  Inputs=*/
  Gain : Gain  Gain=-1/pi
  Gain1 : Gain  Gain=-1
  Max : MinMax  Function=max  Inputs=2
  Max1 : MinMax  Function=max  Inputs=2
  Product : Product
  Product1 : Product  Inputs=3
  Saturation : Saturate  UpperLimit=pi/2  LowerLimit=-pi/2
  Saturation Dynamic : simulink/Discontinuities/Saturation Dynamic  OutMin=[]  OutMax=[]  OutDataTypeStr=Inherit: Same as second input  OutDataType=fixdt(1, 16)  OutScaling=2^-10  DoSatur=off
  deg_2_rad : Gain  Gain=pi / 180
  thermal_derater : Subsystem
  turns_ratio : Gain  Gain=24/15
  i_dab_i : Outport
  i_dab_j : Outport  Port=2
  dab_k : Outport  Port=3
  Temp_Junction : Outport  Port=4
  Temp_HeatSink : Outport  Port=5
  wires:
  Constant/1 -> Max/2, Max1/2
  Add Constant/1 -> Product1/2
  Divide/1 -> Gain1/1
  Max1/1 -> Divide1/2
  Gain1/1 -> i_dab_i/1
  Divide1/1 -> i_dab_j/1
  Saturation Dynamic/1 -> DAB_Thermal_Model/1(P_ij), Divide1/1, Divide/1
  Saturation/1 -> Product1/1, Abs/1
  1/2*pi*fs/1 -> 1/Lk/1
  phase_shift/1 -> deg_2_rad/1
  Gain/1 -> Add Constant/1
  1/Lk/1 -> dab_k/1, Product1/3
  Product/1 -> turns_ratio/1
  turns_ratio/1 -> 1/2*pi*fs/1
  Abs/1 -> Gain/1
  deg_2_rad/1 -> Saturation/1
  Max/1 -> Divide/2
  v_right/1 -> DAB_Thermal_Model/3(Vb), Product/2, Max1/1
  v_left/1 -> DAB_Thermal_Model/2(Va), Max/1, Product/1
  Product1/1 -> Saturation Dynamic/2  "P_ij"
  DAB_Thermal_Model/1(T_j) -> thermal_derater/1(Tj), Temp_Junction/1
  DAB_Thermal_Model/2(T_h) -> Temp_HeatSink/1
  thermal_derater/1(derate_pos) -> Saturation Dynamic/1
  thermal_derater/2(derate_neg) -> Saturation Dynamic/3

== system Grid_modelling_Thermal_V7_ALfix_sheddable_ramped/DAB_Model_CD ==
  phase_shift : Inport
  v_left : Inport  Port=2
  v_right : Inport  Port=3
  1/2*pi*fs : Gain  Gain=1 / (2*pi*10e3)
  1/Lk : Gain  Gain=1 / 340e-6
  Abs : Abs  SaturateOnIntegerOverflow=off
  Add Constant : Bias  Bias=1  SaturateOnIntegerOverflow=off
  Constant : Constant  Value=10
  DAB_Thermal_Model : Subsystem
  Divide : Product  Inputs=*/
  Divide1 : Product  Inputs=*/
  Gain : Gain  Gain=-1/pi
  Gain1 : Gain  Gain=-1
  Max : MinMax  Function=max  Inputs=2
  Max1 : MinMax  Function=max  Inputs=2
  Product : Product
  Product1 : Product  Inputs=3
  Saturation : Saturate  UpperLimit=pi/2  LowerLimit=-pi/2
  Saturation Dynamic : simulink/Discontinuities/Saturation Dynamic  OutMin=[]  OutMax=[]  OutDataTypeStr=Inherit: Same as second input  OutDataType=fixdt(1, 16)  OutScaling=2^-10  DoSatur=off
  Scope : Scope
      settings: ActiveDisplayYMinimum=-12486.00124  ActiveDisplayYMaximum=12374.0112
  deg_2_rad : Gain  Gain=pi / 180
  thermal_derater : Subsystem
  turns_ratio : Gain  Gain=24/15
  i_dab_i : Outport
  i_dab_j : Outport  Port=2
  dab_k : Outport  Port=3
  Temp_Junction : Outport  Port=4
  Temp_HeatSink : Outport  Port=5
  wires:
  Constant/1 -> Max/2, Max1/2
  Add Constant/1 -> Product1/2
  Divide/1 -> Gain1/1
  Max1/1 -> Divide1/2
  Gain1/1 -> i_dab_i/1
  Divide1/1 -> i_dab_j/1
  Saturation Dynamic/1 -> Scope/1, DAB_Thermal_Model/1(P_ij), Divide1/1, Divide/1
  Saturation/1 -> Product1/1, Abs/1
  1/2*pi*fs/1 -> 1/Lk/1
  phase_shift/1 -> deg_2_rad/1
  Gain/1 -> Add Constant/1
  1/Lk/1 -> dab_k/1, Product1/3
  Product/1 -> turns_ratio/1
  turns_ratio/1 -> 1/2*pi*fs/1
  Abs/1 -> Gain/1
  deg_2_rad/1 -> Saturation/1
  Max/1 -> Divide/2
  v_right/1 -> DAB_Thermal_Model/3(Vb), Product/2, Max1/1
  v_left/1 -> DAB_Thermal_Model/2(Va), Max/1, Product/1
  Product1/1 -> Saturation Dynamic/2  "P_ij"
  DAB_Thermal_Model/1(T_j) -> thermal_derater/1(Tj), Temp_Junction/1
  DAB_Thermal_Model/2(T_h) -> Temp_HeatSink/1
  thermal_derater/1(derate_pos) -> Saturation Dynamic/1
  thermal_derater/2(derate_neg) -> Saturation Dynamic/3

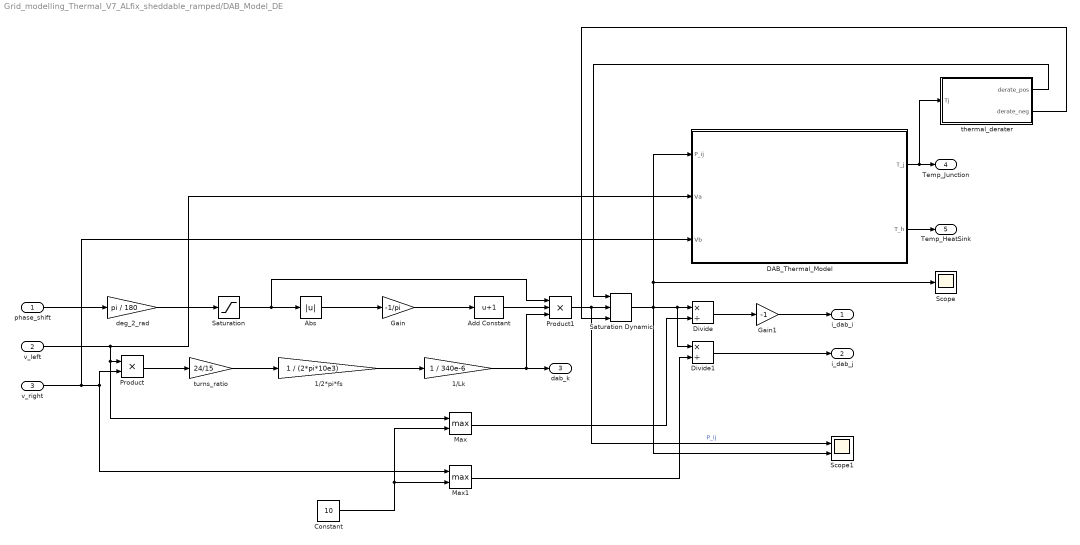
== system Grid_modelling_Thermal_V7_ALfix_sheddable_ramped/DAB_Model_DE ==
  phase_shift : Inport
  v_left : Inport  Port=2
  v_right : Inport  Port=3
  1/2*pi*fs : Gain  Gain=1 / (2*pi*10e3)
  1/Lk : Gain  Gain=1 / 340e-6
  Abs : Abs  SaturateOnIntegerOverflow=off
  Add Constant : Bias  Bias=1  SaturateOnIntegerOverflow=off
  Constant : Constant  Value=10
  DAB_Thermal_Model : Subsystem
  Divide : Product  Inputs=*/
  Divide1 : Product  Inputs=*/
  Gain : Gain  Gain=-1/pi
  Gain1 : Gain  Gain=-1
  Max : MinMax  Function=max  Inputs=2
  Max1 : MinMax  Function=max  Inputs=2
  Product : Product
  Product1 : Product  Inputs=3
  Saturation : Saturate  UpperLimit=pi/2  LowerLimit=-pi/2
  Saturation Dynamic : simulink/Discontinuities/Saturation Dynamic  OutMin=[]  OutMax=[]  OutDataTypeStr=Inherit: Same as second input  OutDataType=fixdt(1, 16)  OutScaling=2^-10  DoSatur=off
  Scope : Scope
      settings: ActiveDisplayYMinimum=-33956.19993  ActiveDisplayYMaximum=3772.9111
  Scope1 : Scope  NumInputPorts=2
      settings: ActiveDisplayYMinimum=-40890.18382  ActiveDisplayYMaximum=4543.35376  DataLoggingVariableName=ScopeData3
  deg_2_rad : Gain  Gain=pi / 180
  thermal_derater : Subsystem
  turns_ratio : Gain  Gain=24/15
  i_dab_i : Outport
  i_dab_j : Outport  Port=2
  dab_k : Outport  Port=3
  Temp_Junction : Outport  Port=4
  Temp_HeatSink : Outport  Port=5
  wires:
  Constant/1 -> Max/2, Max1/2
  Add Constant/1 -> Product1/2
  Divide/1 -> Gain1/1
  Max1/1 -> Divide1/2
  Gain1/1 -> i_dab_i/1
  Divide1/1 -> i_dab_j/1
  Saturation Dynamic/1 -> Scope1/2, Scope/1, DAB_Thermal_Model/1(P_ij), Divide1/1, Divide/1
  Saturation/1 -> Product1/1, Abs/1
  1/2*pi*fs/1 -> 1/Lk/1
  phase_shift/1 -> deg_2_rad/1
  Gain/1 -> Add Constant/1
  1/Lk/1 -> dab_k/1, Product1/3
  Product/1 -> turns_ratio/1
  turns_ratio/1 -> 1/2*pi*fs/1
  Abs/1 -> Gain/1
  deg_2_rad/1 -> Saturation/1
  Max/1 -> Divide/2
  v_right/1 -> DAB_Thermal_Model/3(Vb), Product/2, Max1/1
  v_left/1 -> DAB_Thermal_Model/2(Va), Max/1, Product/1
  Product1/1 -> Saturation Dynamic/2, Scope1/1  "P_ij"
  DAB_Thermal_Model/1(T_j) -> thermal_derater/1(Tj), Temp_Junction/1
  DAB_Thermal_Model/2(T_h) -> Temp_HeatSink/1
  thermal_derater/1(derate_pos) -> Saturation Dynamic/1
  thermal_derater/2(derate_neg) -> Saturation Dynamic/3

== system Grid_modelling_Thermal_V7_ALfix_sheddable_ramped/DAB_Model_EF ==
  phase_shift : Inport
  v_left : Inport  Port=2
  v_right : Inport  Port=3
  1/2*pi*fs : Gain  Gain=1 / (2*pi*10e3)
  1/Lk : Gain  Gain=1 / 340e-6
  Abs : Abs  SaturateOnIntegerOverflow=off
  Add Constant : Bias  Bias=1  SaturateOnIntegerOverflow=off
  Constant : Constant  Value=10
  DAB_Thermal_Model : Subsystem
  Divide : Product  Inputs=*/
  Divide1 : Product  Inputs=*/
  Gain : Gain  Gain=-1/pi
  Gain1 : Gain  Gain=-1
  Max : MinMax  Function=max  Inputs=2
  Max1 : MinMax  Function=max  Inputs=2
  Product : Product
  Product1 : Product  Inputs=3
  Saturation : Saturate  UpperLimit=pi/2  LowerLimit=-pi/2
  Saturation Dynamic : simulink/Discontinuities/Saturation Dynamic  OutMin=[]  OutMax=[]  OutDataTypeStr=Inherit: Same as second input  OutDataType=fixdt(1, 16)  OutScaling=2^-10  DoSatur=off
  deg_2_rad : Gain  Gain=pi / 180
  thermal_derater : Subsystem
  turns_ratio : Gain  Gain=24/15
  i_dab_i : Outport
  i_dab_j : Outport  Port=2
  dab_k : Outport  Port=3
  Temp_Junction : Outport  Port=4
  Temp_HeatSink : Outport  Port=5
  wires:
  Constant/1 -> Max/2, Max1/2
  Add Constant/1 -> Product1/2
  Divide/1 -> Gain1/1
  Max1/1 -> Divide1/2
  Gain1/1 -> i_dab_i/1
  Divide1/1 -> i_dab_j/1
  Saturation Dynamic/1 -> DAB_Thermal_Model/1(P_ij), Divide1/1, Divide/1
  Saturation/1 -> Product1/1, Abs/1
  1/2*pi*fs/1 -> 1/Lk/1
  phase_shift/1 -> deg_2_rad/1
  Gain/1 -> Add Constant/1
  1/Lk/1 -> dab_k/1, Product1/3
  Product/1 -> turns_ratio/1
  turns_ratio/1 -> 1/2*pi*fs/1
  Abs/1 -> Gain/1
  deg_2_rad/1 -> Saturation/1
  Max/1 -> Divide/2
  v_right/1 -> DAB_Thermal_Model/3(Vb), Product/2, Max1/1
  v_left/1 -> DAB_Thermal_Model/2(Va), Max/1, Product/1
  Product1/1 -> Saturation Dynamic/2  "P_ij"
  DAB_Thermal_Model/1(T_j) -> thermal_derater/1(Tj), Temp_Junction/1
  DAB_Thermal_Model/2(T_h) -> Temp_HeatSink/1
  thermal_derater/1(derate_pos) -> Saturation Dynamic/1
  thermal_derater/2(derate_neg) -> Saturation Dynamic/3

== system Grid_modelling_Thermal_V7_ALfix_sheddable_ramped/DAB_Model_FG ==
  phase_shift : Inport
  v_left : Inport  Port=2
  v_right : Inport  Port=3
  1/2*pi*fs : Gain  Gain=1 / (2*pi*10e3)
  1/Lk : Gain  Gain=1 / 340e-6
  Abs : Abs  SaturateOnIntegerOverflow=off
  Add Constant : Bias  Bias=1  SaturateOnIntegerOverflow=off
  Constant : Constant  Value=10
  DAB_Thermal_Model : Subsystem
  Divide : Product  Inputs=*/
  Divide1 : Product  Inputs=*/
  Gain : Gain  Gain=-1/pi
  Gain1 : Gain  Gain=-1
  Max : MinMax  Function=max  Inputs=2
  Max1 : MinMax  Function=max  Inputs=2
  Product : Product
  Product1 : Product  Inputs=3
  Saturation : Saturate  UpperLimit=pi/2  LowerLimit=-pi/2
  Saturation Dynamic : simulink/Discontinuities/Saturation Dynamic  OutMin=[]  OutMax=[]  OutDataTypeStr=Inherit: Same as second input  OutDataType=fixdt(1, 16)  OutScaling=2^-10  DoSatur=off
  deg_2_rad : Gain  Gain=pi / 180
  thermal_derater : Subsystem
  turns_ratio : Gain  Gain=24/15
  i_dab_i : Outport
  i_dab_j : Outport  Port=2
  dab_k : Outport  Port=3
  Temp_Junction : Outport  Port=4
  Temp_HeatSink : Outport  Port=5
  wires:
  Constant/1 -> Max/2, Max1/2
  Add Constant/1 -> Product1/2
  Divide/1 -> Gain1/1
  Max1/1 -> Divide1/2
  Gain1/1 -> i_dab_i/1
  Divide1/1 -> i_dab_j/1
  Saturation Dynamic/1 -> DAB_Thermal_Model/1(P_ij), Divide1/1, Divide/1
  Saturation/1 -> Product1/1, Abs/1
  1/2*pi*fs/1 -> 1/Lk/1
  phase_shift/1 -> deg_2_rad/1
  Gain/1 -> Add Constant/1
  1/Lk/1 -> dab_k/1, Product1/3
  Product/1 -> turns_ratio/1
  turns_ratio/1 -> 1/2*pi*fs/1
  Abs/1 -> Gain/1
  deg_2_rad/1 -> Saturation/1
  Max/1 -> Divide/2
  v_right/1 -> DAB_Thermal_Model/3(Vb), Product/2, Max1/1
  v_left/1 -> DAB_Thermal_Model/2(Va), Max/1, Product/1
  Product1/1 -> Saturation Dynamic/2  "P_ij"
  DAB_Thermal_Model/1(T_j) -> thermal_derater/1(Tj), Temp_Junction/1
  DAB_Thermal_Model/2(T_h) -> Temp_HeatSink/1
  thermal_derater/1(derate_pos) -> Saturation Dynamic/1
  thermal_derater/2(derate_neg) -> Saturation Dynamic/3

== system Grid_modelling_Thermal_V7_ALfix_sheddable_ramped/DAB_Model_GH ==
  phase_shift : Inport
  v_left : Inport  Port=2
  v_right : Inport  Port=3
  1/2*pi*fs : Gain  Gain=1 / (2*pi*10e3)
  1/Lk : Gain  Gain=1 / 340e-6
  Abs : Abs  SaturateOnIntegerOverflow=off
  Add Constant : Bias  Bias=1  SaturateOnIntegerOverflow=off
  Constant : Constant  Value=10
  DAB_Thermal_Model : Subsystem
  Divide : Product  Inputs=*/
  Divide1 : Product  Inputs=*/
  Gain : Gain  Gain=-1/pi
  Gain1 : Gain  Gain=-1
  Max : MinMax  Function=max  Inputs=2
  Max1 : MinMax  Function=max  Inputs=2
  Product : Product
  Product1 : Product  Inputs=3
  Saturation : Saturate  UpperLimit=pi/2  LowerLimit=-pi/2
  Saturation Dynamic : simulink/Discontinuities/Saturation Dynamic  OutMin=[]  OutMax=[]  OutDataTypeStr=Inherit: Same as second input  OutDataType=fixdt(1, 16)  OutScaling=2^-10  DoSatur=off
  deg_2_rad : Gain  Gain=pi / 180
  thermal_derater : Subsystem
  turns_ratio : Gain  Gain=24/15
  i_dab_i : Outport
  i_dab_j : Outport  Port=2
  dab_k : Outport  Port=3
  Temp_Junction : Outport  Port=4
  Temp_HeatSink : Outport  Port=5
  wires:
  Constant/1 -> Max/2, Max1/2
  Add Constant/1 -> Product1/2
  Divide/1 -> Gain1/1
  Max1/1 -> Divide1/2
  Gain1/1 -> i_dab_i/1
  Divide1/1 -> i_dab_j/1
  Saturation Dynamic/1 -> DAB_Thermal_Model/1(P_ij), Divide1/1, Divide/1
  Saturation/1 -> Product1/1, Abs/1
  1/2*pi*fs/1 -> 1/Lk/1
  phase_shift/1 -> deg_2_rad/1
  Gain/1 -> Add Constant/1
  1/Lk/1 -> dab_k/1, Product1/3
  Product/1 -> turns_ratio/1
  turns_ratio/1 -> 1/2*pi*fs/1
  Abs/1 -> Gain/1
  deg_2_rad/1 -> Saturation/1
  Max/1 -> Divide/2
  v_right/1 -> DAB_Thermal_Model/3(Vb), Product/2, Max1/1
  v_left/1 -> DAB_Thermal_Model/2(Va), Max/1, Product/1
  Product1/1 -> Saturation Dynamic/2  "P_ij"
  DAB_Thermal_Model/1(T_j) -> thermal_derater/1(Tj), Temp_Junction/1
  DAB_Thermal_Model/2(T_h) -> Temp_HeatSink/1
  thermal_derater/1(derate_pos) -> Saturation Dynamic/1
  thermal_derater/2(derate_neg) -> Saturation Dynamic/3

== system Grid_modelling_Thermal_V7_ALfix_sheddable_ramped/DAB_Model_HK ==
  phase_shift : Inport
  v_left : Inport  Port=2
  v_right : Inport  Port=3
  1/2*pi*fs : Gain  Gain=1 / (2*pi*10e3)
  1/Lk : Gain  Gain=1 / 340e-6
  Abs : Abs  SaturateOnIntegerOverflow=off
  Add Constant : Bias  Bias=1  SaturateOnIntegerOverflow=off
  Constant : Constant  Value=10
  DAB_Thermal_Model : Subsystem
  Divide : Product  Inputs=*/
  Divide1 : Product  Inputs=*/
  Gain : Gain  Gain=-1/pi
  Gain1 : Gain  Gain=-1
  Max : MinMax  Function=max  Inputs=2
  Max1 : MinMax  Function=max  Inputs=2
  Product : Product
  Product1 : Product  Inputs=3
  Saturation : Saturate  UpperLimit=pi/2  LowerLimit=-pi/2
  Saturation Dynamic : simulink/Discontinuities/Saturation Dynamic  OutMin=[]  OutMax=[]  OutDataTypeStr=Inherit: Same as second input  OutDataType=fixdt(1, 16)  OutScaling=2^-10  DoSatur=off
  deg_2_rad : Gain  Gain=pi / 180
  thermal_derater : Subsystem
  turns_ratio : Gain  Gain=24/15
  i_dab_i : Outport
  i_dab_j : Outport  Port=2
  dab_k : Outport  Port=3
  Temp_Junction : Outport  Port=4
  Temp_HeatSink : Outport  Port=5
  wires:
  Constant/1 -> Max/2, Max1/2
  Add Constant/1 -> Product1/2
  Divide/1 -> Gain1/1
  Max1/1 -> Divide1/2
  Gain1/1 -> i_dab_i/1
  Divide1/1 -> i_dab_j/1
  Saturation Dynamic/1 -> DAB_Thermal_Model/1(P_ij), Divide1/1, Divide/1
  Saturation/1 -> Product1/1, Abs/1
  1/2*pi*fs/1 -> 1/Lk/1
  phase_shift/1 -> deg_2_rad/1
  Gain/1 -> Add Constant/1
  1/Lk/1 -> dab_k/1, Product1/3
  Product/1 -> turns_ratio/1
  turns_ratio/1 -> 1/2*pi*fs/1
  Abs/1 -> Gain/1
  deg_2_rad/1 -> Saturation/1
  Max/1 -> Divide/2
  v_right/1 -> DAB_Thermal_Model/3(Vb), Product/2, Max1/1
  v_left/1 -> DAB_Thermal_Model/2(Va), Max/1, Product/1
  Product1/1 -> Saturation Dynamic/2  "P_ij"
  DAB_Thermal_Model/1(T_j) -> thermal_derater/1(Tj), Temp_Junction/1
  DAB_Thermal_Model/2(T_h) -> Temp_HeatSink/1
  thermal_derater/1(derate_pos) -> Saturation Dynamic/1
  thermal_derater/2(derate_neg) -> Saturation Dynamic/3

== system Grid_modelling_Thermal_V7_ALfix_sheddable_ramped/DAB_Model_KL ==
  phase_shift : Inport
  v_left : Inport  Port=2
  v_right : Inport  Port=3
  1/2*pi*fs : Gain  Gain=1 / (2*pi*10e3)
  1/Lk : Gain  Gain=1 / 340e-6
  Abs : Abs  SaturateOnIntegerOverflow=off
  Add Constant : Bias  Bias=1  SaturateOnIntegerOverflow=off
  Constant : Constant  Value=10
  DAB_Thermal_Model : Subsystem
  Divide : Product  Inputs=*/
  Divide1 : Product  Inputs=*/
  Gain : Gain  Gain=-1/pi
  Gain1 : Gain  Gain=-1
  Max : MinMax  Function=max  Inputs=2
  Max1 : MinMax  Function=max  Inputs=2
  Product : Product
  Product1 : Product  Inputs=3
  Saturation : Saturate  UpperLimit=pi/2  LowerLimit=-pi/2
  Saturation Dynamic : simulink/Discontinuities/Saturation Dynamic  OutMin=[]  OutMax=[]  OutDataTypeStr=Inherit: Same as second input  OutDataType=fixdt(1, 16)  OutScaling=2^-10  DoSatur=off
  deg_2_rad : Gain  Gain=pi / 180
  thermal_derater : Subsystem
  turns_ratio : Gain  Gain=24/15
  i_dab_i : Outport
  i_dab_j : Outport  Port=2
  dab_k : Outport  Port=3
  Temp_Junction : Outport  Port=4
  Temp_HeatSink : Outport  Port=5
  wires:
  Constant/1 -> Max/2, Max1/2
  Add Constant/1 -> Product1/2
  Divide/1 -> Gain1/1
  Max1/1 -> Divide1/2
  Gain1/1 -> i_dab_i/1
  Divide1/1 -> i_dab_j/1
  Saturation Dynamic/1 -> DAB_Thermal_Model/1(P_ij), Divide1/1, Divide/1
  Saturation/1 -> Product1/1, Abs/1
  1/2*pi*fs/1 -> 1/Lk/1
  phase_shift/1 -> deg_2_rad/1
  Gain/1 -> Add Constant/1
  1/Lk/1 -> dab_k/1, Product1/3
  Product/1 -> turns_ratio/1
  turns_ratio/1 -> 1/2*pi*fs/1
  Abs/1 -> Gain/1
  deg_2_rad/1 -> Saturation/1
  Max/1 -> Divide/2
  v_right/1 -> DAB_Thermal_Model/3(Vb), Product/2, Max1/1
  v_left/1 -> DAB_Thermal_Model/2(Va), Max/1, Product/1
  Product1/1 -> Saturation Dynamic/2  "P_ij"
  DAB_Thermal_Model/1(T_j) -> thermal_derater/1(Tj), Temp_Junction/1
  DAB_Thermal_Model/2(T_h) -> Temp_HeatSink/1
  thermal_derater/1(derate_pos) -> Saturation Dynamic/1
  thermal_derater/2(derate_neg) -> Saturation Dynamic/3

== system Grid_modelling_Thermal_V7_ALfix_sheddable_ramped/source_bus_model_A ==
  Pload : Inport
  i_dab_1 : Inport  Port=2
  i_dab_2 : Inport  Port=3
  1/C_bus : Gain  Gain=1/0.01
  1/Rsrc_k : Gain  Gain=1/(0.32*1)
  Add : Sum  Inputs=+-++
  Bus_Bar_Thermal_Model : Subsystem
  Constant : Constant  Value=0
  Divide : Product  Inputs=*/
  Divide1 : Product  Inputs=*/
  I_max : Constant  Value=125
  Integrator : Integrator  InitialCondition=800  LimitOutput=on  LowerSaturationLimit=0
  Max : MinMax  Function=max  Inputs=2
  Max1 : MinMax  Function=max  Inputs=2
  Max2 : MinMax  Function=max  Inputs=2
  Min : MinMax  Inputs=2
  Min1 : MinMax  Inputs=2
  P_max : Constant  Value=100e3
  Product : Product
  Subtract : Sum  Inputs=+-
  V_th_k : Constant  Value=800
  div_by_zero_protect : Constant  Value=10
  div_by_zero_protect1 : Constant  Value=10
  V_bus : Outport
  Bus_Power : Outport  Port=2
  Temp_bus : Outport  Port=3
  wires:
  Max2/1 -> Divide1/2
  Divide/1 -> Min1/2  "i_pmax_k"
  1/Rsrc_k/1 -> Max/1  "i_th_k"
  Min/1 -> Min1/1  "i_lim_k"
  Subtract/1 -> 1/Rsrc_k/1
  Add/1 -> 1/C_bus/1
  1/C_bus/1 -> Integrator/1
  Integrator/1 -> Product/1, V_bus/1, Max2/1, Max1/1, Subtract/2
  Divide1/1 -> Add/2
  V_th_k/1 -> Subtract/1
  Pload/1 -> Divide1/1
  Constant/1 -> Max/2
  Max/1 -> Min/1
  i_dab_1/1 -> Add/3
  I_max/1 -> Min/2
  Min1/1 -> Add/1, Bus_Bar_Thermal_Model/1(i_src_k), Product/2  "i_src_k"
  P_max/1 -> Divide/1
  Max1/1 -> Divide/2
  i_dab_2/1 -> Add/4
  div_by_zero_protect1/1 -> Max2/2
  div_by_zero_protect/1 -> Max1/2
  Product/1 -> Bus_Power/1
  Bus_Bar_Thermal_Model/1(T_bus) -> Temp_bus/1

== system Grid_modelling_Thermal_V7_ALfix_sheddable_ramped/source_bus_model_B ==
  Pload : Inport
  i_dab_1 : Inport  Port=2
  i_dab_2 : Inport  Port=3
  1/C_bus : Gain  Gain=1/0.01
  Add : Sum  Inputs=+-++
  Bus_Bar_Thermal_Model : Subsystem
  Constant : Constant  Value=0
  Divide : Product  Inputs=*/
  Divide1 : Product  Inputs=*/
  I_max : Constant  Value=125
  Integrator : Integrator  InitialCondition=800  LimitOutput=on  LowerSaturationLimit=0
  Max : MinMax  Function=max  Inputs=2
  Max1 : MinMax  Function=max  Inputs=2
  Max2 : MinMax  Function=max  Inputs=2
  Min : MinMax  Inputs=2
  Min1 : MinMax  Inputs=2
  P_max : Constant  Value=100e3
  Product : Product
  Product1 : Product
  Step : Step  Time=1000  Before=1 / (0.32*1)  After=1 / (0.32*1)  SampleTime=0
  Subtract : Sum  Inputs=+-
  V_th_k : Constant  Value=800
  div_by_zero_protect : Constant  Value=10
  div_by_zero_protect1 : Constant  Value=10
  V_bus : Outport
  Bus_Power : Outport  Port=2
  Temp_bus : Outport  Port=3
  wires:
  Max2/1 -> Divide1/2
  Divide/1 -> Min1/2  "i_pmax_k"
  Product1/1 -> Max/1  "i_th_k"
  Min/1 -> Min1/1  "i_lim_k"
  Subtract/1 -> Product1/2
  Add/1 -> 1/C_bus/1
  1/C_bus/1 -> Integrator/1
  Divide1/1 -> Add/2
  V_th_k/1 -> Subtract/1
  Pload/1 -> Divide1/1
  Constant/1 -> Max/2
  Max/1 -> Min/1
  i_dab_1/1 -> Add/3
  I_max/1 -> Min/2
  P_max/1 -> Divide/1
  Max1/1 -> Divide/2
  i_dab_2/1 -> Add/4
  div_by_zero_protect1/1 -> Max2/2
  div_by_zero_protect/1 -> Max1/2
  Integrator/1 -> Product/1, V_bus/1, Max2/1, Max1/1, Subtract/2
  Product/1 -> Bus_Power/1
  Min1/1 -> Bus_Bar_Thermal_Model/1(i_src_k), Product/2, Add/1  "i_src_k"
  Bus_Bar_Thermal_Model/1(T_bus) -> Temp_bus/1
  Step/1 -> Product1/1

== system Grid_modelling_Thermal_V7_ALfix_sheddable_ramped/source_bus_model_C ==
  Pload : Inport
  i_dab_1 : Inport  Port=2
  i_dab_2 : Inport  Port=3
  1/C_bus : Gain  Gain=1/0.01
  Add : Sum  Inputs=+-++
  Bus_Bar_Thermal_Model : Subsystem
  Constant : Constant  Value=0
  Divide : Product  Inputs=*/
  Divide1 : Product  Inputs=*/
  I_max : Constant  Value=125
  Integrator : Integrator  InitialCondition=800  LimitOutput=on  LowerSaturationLimit=0
  Max : MinMax  Function=max  Inputs=2
  Max1 : MinMax  Function=max  Inputs=2
  Max2 : MinMax  Function=max  Inputs=2
  Min : MinMax  Inputs=2
  Min1 : MinMax  Inputs=2
  P_max : Constant  Value=100e3
  Product : Product
  Product1 : Product
  Step : Step  Time=2250  Before=1 / (0.32*1)  After=1 / (0.32*1)  SampleTime=0
  Subtract : Sum  Inputs=+-
  V_th_k : Constant  Value=800
  div_by_zero_protect : Constant  Value=10
  div_by_zero_protect1 : Constant  Value=10
  V_bus : Outport
  Bus_Power : Outport  Port=2
  Temp_bus : Outport  Port=3
  wires:
  Max2/1 -> Divide1/2
  Divide/1 -> Min1/2  "i_pmax_k"
  Product1/1 -> Max/1  "i_th_k"
  Min/1 -> Min1/1  "i_lim_k"
  Subtract/1 -> Product1/2
  Add/1 -> 1/C_bus/1
  1/C_bus/1 -> Integrator/1
  Divide1/1 -> Add/2
  V_th_k/1 -> Subtract/1
  Pload/1 -> Divide1/1
  Constant/1 -> Max/2
  Max/1 -> Min/1
  i_dab_1/1 -> Add/3
  I_max/1 -> Min/2
  P_max/1 -> Divide/1
  Max1/1 -> Divide/2
  i_dab_2/1 -> Add/4
  div_by_zero_protect1/1 -> Max2/2
  div_by_zero_protect/1 -> Max1/2
  Integrator/1 -> Product/1, V_bus/1, Max2/1, Max1/1, Subtract/2
  Product/1 -> Bus_Power/1
  Min1/1 -> Bus_Bar_Thermal_Model/1(i_src_k), Product/2, Add/1  "i_src_k"
  Bus_Bar_Thermal_Model/1(T_bus) -> Temp_bus/1
  Step/1 -> Product1/1
